simulink model "Simfinal"  (R2026a)
settings: Solver=VariableStepAuto
undefined symbols (not defined in the file): B, dspblkCoreblockFVToolHelper, gcbh, J, K, Ka, L, q0, q1, q2, R, s0, tm
settings Model: Creator=jusem  LastModifiedBy=jusem

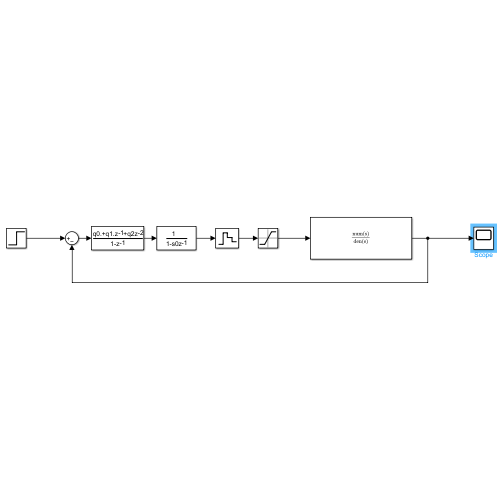
[thumbnail: Simulink's stored preview of the top-level diagram]
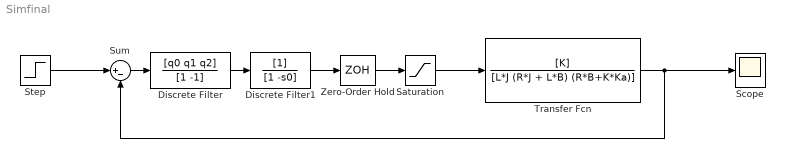
== system Simfinal ==
  Discrete Filter : DiscreteFilter  LoadFcn=dspblkCoreblockFVToolHelper(gcbh,'load');  Numerator=[q0 q1 q2]  Denominator=[1 -1]
      settings: CopyFcn=dspblkCoreblockFVToolHelper(gcbh,'copy');  DeleteFcn=dspblkCoreblockFVToolHelper(gcbh,'close');  ModelCloseFcn=dspblkCoreblockFVToolHelper(gcbh,'close');  PreSaveFcn=dspblkCoreblockFVToolHelper(gcbh,'presave');  PostSaveFcn=dspblkCoreblockFVToolHelper(gcbh,'postsave');  CloseFcn=dspblkCoreblockFVToolHelper(gcbh,'close');
  Discrete Filter1 : DiscreteFilter  LoadFcn=dspblkCoreblockFVToolHelper(gcbh,'load');  Denominator=[1 -s0]
      settings: CopyFcn=dspblkCoreblockFVToolHelper(gcbh,'copy');  DeleteFcn=dspblkCoreblockFVToolHelper(gcbh,'close');  ModelCloseFcn=dspblkCoreblockFVToolHelper(gcbh,'close');  PreSaveFcn=dspblkCoreblockFVToolHelper(gcbh,'presave');  PostSaveFcn=dspblkCoreblockFVToolHelper(gcbh,'postsave');  CloseFcn=dspblkCoreblockFVToolHelper(gcbh,'close');
  Saturation : Saturate  UpperLimit=12  LowerLimit=-12
  Scope : Scope
      settings: ActiveDisplayYMinimum=-3.3848352677831524  ActiveDisplayYMaximum=5.9316483630870165
  Step : Step  FinalValue=5  SampleTime=0
  Sum : Sum  Inputs=|+-
  Transfer Fcn : TransferFcn  Numerator=[K]  Denominator=[L*J (R*J + L*B) (R*B+K*Ka)]
  Zero-Order Hold : ZeroOrderHold  SampleTime=tm
  wires:
  Step/1 -> Sum/1
  Sum/1 -> Discrete Filter/1
  Zero-Order Hold/1 -> Saturation/1
  Transfer Fcn/1 -> Scope/1, Sum/2
  Discrete Filter/1 -> Discrete Filter1/1
  Discrete Filter1/1 -> Zero-Order Hold/1
  Saturation/1 -> Transfer Fcn/1
